simulink model "Exp4"  (R2025b)
settings: Solver=VariableStepAuto  StartTime=0.0  StopTime=10  RelTol=1e-3
libraries: dspstat3 x2, dspsrcs4 x2
settings Model: Creator=pc  LastModifiedBy=pc

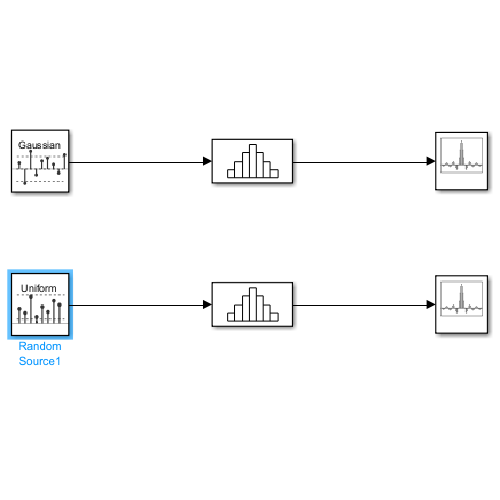
[thumbnail: Simulink's stored preview of the top-level diagram]
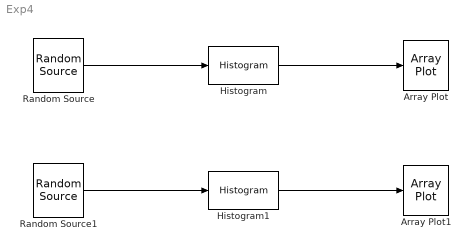
== system Exp4 ==
  Array Plot : ArrayPlot  WindowPosition=[283.000000,134.000000,800.000000,500.000000,]  ScopeFrameLocation=window  YLimits=[-993.25 8939.25]
  Array Plot1 : ArrayPlot  WindowPosition=[283.000000,134.000000,800.000000,500.000000,]  ScopeFrameLocation=window  YLimits=[-2515.125 22636.125]
  Histogram : dspstat3/Histogram  umin=-5  umax=5  nbins=50  operateOver=Each column  Dimension=1  normalized=off  run=off  reset=on  trigtype=Non-zero sample  colComp=on  roundingMode=Floor  overflowMode=off  accumDataTypeStr=Inherit: Same as product output  accumLastDataTypeStr=Inherit: Same as product output
  Histogram1 : dspstat3/Histogram  umin=-5  umax=5  nbins=50  operateOver=Each column  Dimension=1  normalized=off  run=off  reset=on  trigtype=Non-zero sample  colComp=on  roundingMode=Floor  overflowMode=off  accumDataTypeStr=Inherit: Same as product output  accumLastDataTypeStr=Inherit: Same as product output
  Random Source : dspsrcs4/Random Source  SrcType=Gaussian  MinVal=0  MaxVal=1  MeanVal=0  VarVal=1  RepMode=Specify seed  rawSeed=1  IsInherit=off  SampTime=1  SampFrame=100000  OutComplex=Real  DataType=double  SimulateUsing=Interpreted execution
  Random Source1 : dspsrcs4/Random Source  SrcType=Uniform  MinVal=0  MaxVal=1  MeanVal=0  VarVal=1  RepMode=Specify seed  rawSeed=1  IsInherit=off  SampTime=1  SampFrame=100000  OutComplex=Real  DataType=double  SimulateUsing=Interpreted execution
  wires:
  Random Source/1 -> Histogram/1
  Histogram/1 -> Array Plot/1
  Random Source1/1 -> Histogram1/1
  Histogram1/1 -> Array Plot1/1
